simulink model "Modelo_control_d_2GDL_2021"  (R2021b)
settings: Solver=ode45  StartTime=0.0  StopTime=10
values from neighbouring files (symbols this model uses):
  airgap = r.air_gap/1000    [initializationControl.m]
  current_I = r.current(1,2:32)    [initializationControl.m]
  currentSensorNoise = 0.06^2    (= 0.0036)    [initializationControl.m]
  dtCurrent = 1e-4    (= 0.0001)    [initializationControl.m]
  dTSensor = 5e-4    (= 0.0005)    [initializationControl.m]
  filterConstant = 30    [initializationControl.m]
  inductance = r.inductance    [initializationControl.m]
  K_d = place(Ad2,Bd2,polos_dis)    [initializationControl.m]
  Ki = 100    [initializationControl.m]
  Kp = 25    [initializationControl.m]
  m = pod.mass.mass    [initializationControl.m]
  noiseSensor = 0.05*1e-3    (= 5e-05)    [initializationControl.m]
  Rcoil = 0.242    [initializationControl.m]
  resCurrent = 156.11/7200    (= 0.0216819444444)    [initializationControl.m]
  s = tf('s')    [initializationControl.m]
  T = 0.001    [initializationControl.m]
  tauFilterCurrent = 0.001    [initializationControl.m]
  thetafilter = 40    [initializationControl.m]
  z_0 = 18e-3    (= 0.018)    [initializationControl.m]
  z_ini = z_0 + z_lev    [initializationControl.m]
  z_lev = pod.geometry.z_LEV    [initializationControl.m]
undefined symbols (not defined in the file or in its folder): DiscIntNeverNeededParam, h, initial_conds, km, pod
libraries: cstblocks x5, slpidlib x3, aerolibconvert2 x1
(part 2 of 2)

== matlab function Modelo_control_d_2GDL_2021/Modelo no-lineal/Non-linear 3 DOF model/H7 Pod Dynamic model (3DOF)/LIM/MATLAB Function2 ==
  data: v input; x input; sign output; pod parameter
function sign = LIMdirection(v, x, pod)
% Decides if the LIM force is being applied to accelerate or to brake 
% by comparing the position of the pod with a predefined treshold
% ═════════════════════════════════════════════════════════════════════════
% Last updated: 20.12.2021
% ═════════════════════════════════════════════════════════════════════════


if x >= pod.brakes.lim_off 
    sign = 0;
elseif x < pod.brakes.lim_off && x >= pod.brakes.lim_brake && v > 0    
    sign = -1;
else
    sign = 1;
end

== matlab function Modelo_control_d_2GDL_2021/Modelo no-lineal/Non-linear 3 DOF model/H7 Pod Dynamic model (3DOF)/LIM/MATLAB Function ==
  data: v input; acceleration_flag input; F output; pod parameter
function F = LIMtraction(v, acceleration_flag, pod)
% Computes the traction force (N) of the LIM as a function of 
% the absolute velocity of the prototype (m/s)
% ═════════════════════════════════════════════════════════════════════════
% Last updated: 20.12.2021
% ═════════════════════════════════════════════════════════════════════════

if acceleration_flag == 1
    F = pod.propulsion.poly.p3*v^3 + ...
        pod.propulsion.poly.p2*v^2 + ...
        pod.propulsion.poly.p1*v   + ...
        pod.propulsion.poly.p0;
else
    F = (pod.propulsion.br_poly.p2*v^2 + ...
        pod.propulsion.br_poly.p1*v   + ...
        pod.propulsion.br_poly.p0);
end

== matlab function Modelo_control_d_2GDL_2021/Modelo no-lineal/Non-linear 3 DOF model/H7 Pod Dynamic model (3DOF)/LIM/MATLAB Function1 ==
  data: v input; v_1 input; x input; sign output; pod parameter; flag output
function [sign, flag] = LIMdirection(v, v_1, x, pod)
% Decides if the LIM force is being applied to accelerate or to brake 
% by comparing the position of the pod with a predefined treshold
% ═════════════════════════════════════════════════════════════════════════
% Last updated: 20.12.2021
% ═════════════════════════════════════════════════════════════════════════

% Acceleration: 1
% Brake: -1
% Otherwise: 0

sign = 0;
% tol = 1e-4;

if v - v_1 > 0
    flag = 1;
elseif v - v_1 < 0
    flag = -1;
else
    flag = 0;
end

if x >= pod.brakes.lim_brake && v >= 0    
    sign = -1;
end

if flag == -1 && v <= pod.brakes.v_max
    sign = 0;
end

if flag ~= -1 && x < pod.brakes.lim_brake
    sign = 1;
end

== matlab function Modelo_control_d_2GDL_2021/Modelo no-lineal/Non-linear 3 DOF model/H7 Pod Dynamic model (3DOF)/Brakes /MATLAB Function ==
  data: x input; velocity input; F output; emergency input; pod parameter
function F  = brakes_activation(x, velocity, emergency, pod)
% Computes the braking force of the pneumatic actuators if and only if 
%     (1) The emergency flag has been raised
%     (2) The pod is above the acceleration phase distance
% ═════════════════════════════════════════════════════════════════════════
% Last updated: 20.12.2021
% ═════════════════════════════════════════════════════════════════════════

num_brakes = pod.brakes.n;

if (emergency == 1 && x >= pod.brakes.d && velocity >= 0)
    F       = pod.brakes.force * ones(num_brakes,1);
else
    F       = zeros(num_brakes,1);
end

== matlab function Modelo_control_d_2GDL_2021/Modelo no-lineal/Non-linear 3 DOF model/H7 Pod Dynamic model (3DOF)/LIM /MATLAB Function ==
  data: v input; F output; pod parameter
function F = LIMtraction(v, pod)
% Computes the traction force (N) of the LIM as a function of 
% the absolute velocity of the prototype (m/s)
% ═════════════════════════════════════════════════════════════════════════
% Last updated: 20.12.2021
% ═════════════════════════════════════════════════════════════════════════

F = pod.propulsion.poly.p3*v^3 + ...
    pod.propulsion.poly.p2*v^2 + ...
    pod.propulsion.poly.p1*v   + ...
    pod.propulsion.poly.p0;

== matlab function Modelo_control_d_2GDL_2021/Modelo no-lineal/Non-linear 3 DOF model/H7 Pod Dynamic model (3DOF)/LIM /MATLAB Function1 ==
  data: v input; x input; sign output; pod parameter
function sign = LIMdirection(v, x, pod)
% Decides if the LIM force is being applied to accelerate or to brake 
% by comparing the position of the pod with a predefined treshold
% ═════════════════════════════════════════════════════════════════════════
% Last updated: 20.12.2021
% ═════════════════════════════════════════════════════════════════════════

if x >= pod.brakes.d && v > 0    
    sign = -1;
elseif x >= pod.brakes.d && v <= 0
    sign = 0;
else
    sign = 1;
end

== matlab function Modelo_control_d_2GDL_2021/Modelo no-lineal/Non-linear 3 DOF model/H7 Pod Dynamic model (3DOF)/Levitation /MATLAB Function ==
  data: v input; F output; pod parameter
function F = HEMSdrag(v, pod)
% Computes the drag force (N) of one HEMS unit as a function of the 
% velocity (m/s)
% ═════════════════════════════════════════════════════════════════════════
% Last updated: 16.01.2022
% ═════════════════════════════════════════════════════════════════════════

if v < 1e-3
    v = 0;
end

F = pod.levitation.drag_1_unit.poly.p3*v^3 + ...
    pod.levitation.drag_1_unit.poly.p2*v^2 + ...
    pod.levitation.drag_1_unit.poly.p1*v   + ...
    pod.levitation.drag_1_unit.poly.p0;

== matlab function Modelo_control_d_2GDL_2021/Modelo no-lineal/Non-linear 3 DOF model/H7 Pod Dynamic model (3DOF)/Levitation /MATLAB Function1 ==
  data: airgap input; F output; intensity input; pod parameter
function F = HEMSlev(airgap, intensity, pod)
% Computes the levitation force (N) of all the HEMS units as a function of 
% their air gaps (mm) and intensities (A)
% ═════════════════════════════════════════════════════════════════════════
% Last updated: 15.12.2021
% ════════════════════════════════════════════════════════════════════════

x   = airgap;
y   = intensity;

F = pod.levitation.poly_1_unit.p00 + ...
    pod.levitation.poly_1_unit.p10.*x + ...
    pod.levitation.poly_1_unit.p01.*y + ...
    pod.levitation.poly_1_unit.p20.*x.^2 + ...
    pod.levitation.poly_1_unit.p11.*x.*y + ...
    pod.levitation.poly_1_unit.p02.*y.^2 + ...
    pod.levitation.poly_1_unit.p21.*x.^2.*y + ...
    pod.levitation.poly_1_unit.p12.*x.*y.^2 + ...
    pod.levitation.poly_1_unit.p03.*y.^3;
